simulink model "PIDantiwindup"  (Simulink 7.1)
settings: Solver=ode45  StartTime=0.0  StopTime=10.0  RelTol=1e-3
undefined symbols (not defined in the file): Kp, Td, Ti
settings Model: Creator=Paul Acquatella  LastModifiedBy=Paul Acquatella

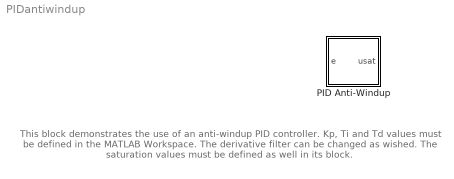
== system PIDantiwindup ==
  note: This block demonstrates the use of an anti-windup PID controller.
      | Kp, Ti and Td values must be defined in the MATLAB Workspace.
      | The derivative filter can be changed as wished.
      | The saturation values must be defined as well in its block.
  PID Anti-Windup : Subsystem

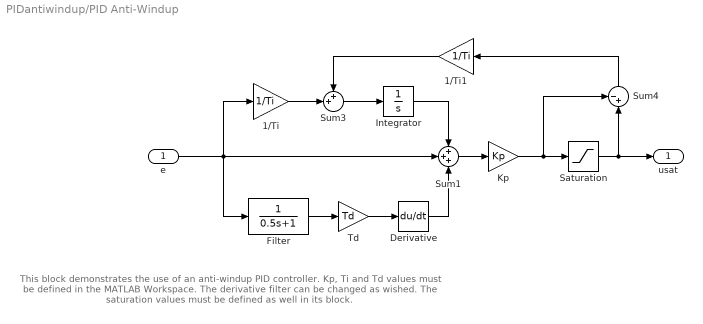
== system PIDantiwindup/PID Anti-Windup ==
  note: This block demonstrates the use of an anti-windup PID controller.
      | Kp, Ti and Td values must be defined in the MATLAB Workspace.
      | The derivative filter can be changed as wished.
      | The saturation values must be defined as well in its block.
  e : Inport  OutDataType=sfix(16)  OutScaling=2^0
  1/Ti : Gain  Gain=1/Ti  ParameterDataType=sfix(16)  ParameterScaling=2^0  OutDataType=sfix(16)  OutScaling=2^0
  1/Ti1 : Gain  Orientation=left  Gain=1/Ti  ParameterDataType=sfix(16)  ParameterScaling=2^0  OutDataType=sfix(16)  OutScaling=2^0
  Derivative : Derivative
  Filter : TransferFcn  Denominator=[0.5 1]
  Integrator : Integrator
  Kp : Gain  Gain=Kp  ParameterDataType=sfix(16)  ParameterScaling=2^0  OutDataType=sfix(16)  OutScaling=2^0
  Saturation : Saturate  UpperLimit=10  LowerLimit=0  OutDataType=sfix(16)  OutScaling=2^0
  Sum1 : Sum  Inputs=+++  OutDataType=sfix(16)  OutScaling=2^0
  Sum3 : Sum  Inputs=++|  OutDataType=sfix(16)  OutScaling=2^0
  Sum4 : Sum  Orientation=up  Inputs=-+|  OutDataType=sfix(16)  OutScaling=2^0
  Td : Gain  Gain=Td  ParameterDataType=sfix(16)  ParameterScaling=2^0  OutDataType=sfix(16)  OutScaling=2^0
  usat : Outport  OutDataType=sfix(16)  OutScaling=2^0
  wires:
  1/Ti1/1 -> Sum3/1
  Sum3/1 -> Integrator/1
  1/Ti/1 -> Sum3/2
  Kp/1 -> Saturation/1, Sum4/1
  Integrator/1 -> Sum1/1
  Saturation/1 -> usat/1, Sum4/2
  Derivative/1 -> Sum1/3
  Sum1/1 -> Kp/1
  e/1 -> Sum1/2, 1/Ti/1, Filter/1
  Td/1 -> Derivative/1
  Filter/1 -> Td/1
  Sum4/1 -> 1/Ti1/1
